simulink model "simulation"  (R2024b)
settings: Solver=VariableStepAuto  StartTime=0.0  StopTime=10.0  RelTol=1e-3
undefined symbols (not defined in the file or in its folder): G, H
settings Model: Creator=muradaliyev  LastModifiedBy=muradaliyev

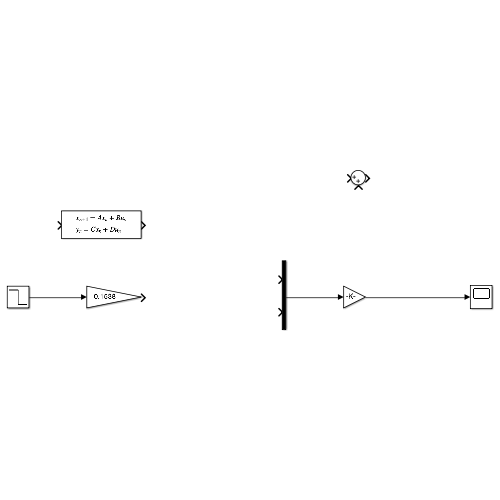
[thumbnail: Simulink's stored preview of the top-level diagram]
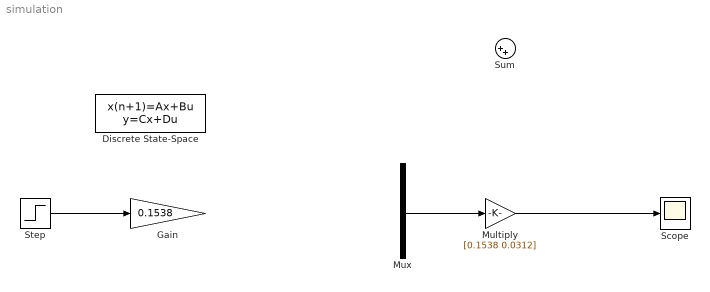
== system simulation ==
  Discrete State-Space : DiscreteStateSpace  A=G  B=H  C=[1 0]  D=0  SampleTime=0.01
  Gain : Gain  Gain=0.1538
  Multiply : Gain  Gain=[0.1538 0.0312]
  Mux : Mux  Inputs=2
  Scope : Scope
  Step : Step  Time=0  Before=10  SampleTime=0
  Sum : Sum  Inputs=|++
  wires:
  Step/1 -> Gain/1
  Mux/1 -> Multiply/1
  Multiply/1 -> Scope/1
